simulink model "final_project_dscrt_agmnt"  (R2019b)
settings: Solver=FixedStepAuto  StartTime=0.0  StopTime=10.0  FixedStep=0.01  RelTol=1e-3
undefined symbols (not defined in the file or in its folder): DiscIntNeverNeededParam
libraries: fuzblock x3, simulink x1
settings Model: Creator=Mertcan  LastModifiedBy=Mertcan

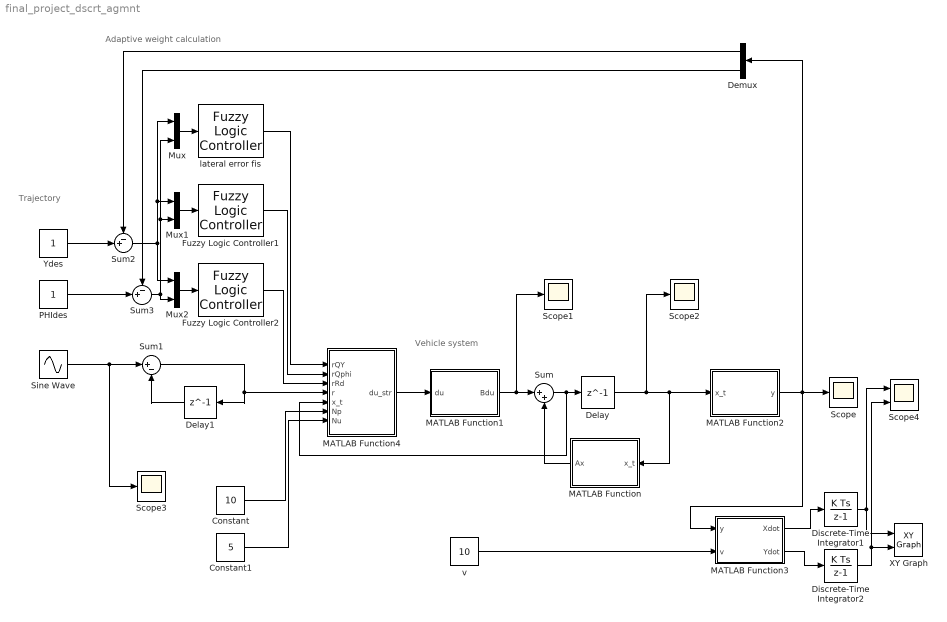
== system final_project_dscrt_agmnt ==
  note: Trajectory
  note: Vehicle system
  note: Adaptive weight calculation
  Constant : Constant  Value=10
  Constant1 : Constant  Value=5
  Delay : Delay  DelayLength=1  SampleTime=0.01
  Delay1 : Delay  DelayLength=1  SampleTime=0.01
  Demux : Demux  Outputs=2
  Discrete-Time Integrator1 : DiscreteIntegrator  SampleTime=0.01  ICPrevOutput=DiscIntNeverNeededParam  ICPrevScaledInput=DiscIntNeverNeededParam
  Discrete-Time Integrator2 : DiscreteIntegrator  SampleTime=0.01  ICPrevOutput=DiscIntNeverNeededParam  ICPrevScaledInput=DiscIntNeverNeededParam
  Fuzzy Logic Controller1 : fuzblock/Fuzzy Logic  Controller  FIS='head_err_surf.fis'  OutputSampleNumber=101  DataType=double  FuzzifiedInputs=off  RuleFiringStrengths=off  RuleOutputs=off  AggregatedOutputs=off  SimulateUsing=Interpreted execution  OutOfRangeInputValueMessage=warning  NoRuleFiredMessage=warning  EmptyOutputFuzzySetMessage=warning
  Fuzzy Logic Controller2 : fuzblock/Fuzzy Logic  Controller  FIS='ang_inc_fw.fis'  OutputSampleNumber=101  DataType=double  FuzzifiedInputs=off  RuleFiringStrengths=off  RuleOutputs=off  AggregatedOutputs=off  SimulateUsing=Interpreted execution  OutOfRangeInputValueMessage=warning  NoRuleFiredMessage=warning  EmptyOutputFuzzySetMessage=warning
  MATLAB Function : MATLAB Function  TreatAsAtomicUnit=on
  MATLAB Function1 : MATLAB Function  TreatAsAtomicUnit=on
  MATLAB Function2 : MATLAB Function  TreatAsAtomicUnit=on
  MATLAB Function3 : MATLAB Function  TreatAsAtomicUnit=on
  MATLAB Function4 : MATLAB Function  TreatAsAtomicUnit=on
  Mux : Mux  Inputs=2
  Mux1 : Mux  Inputs=2
  Mux2 : Mux  Inputs=2
  PHIdes : Constant
  Scope{,1..3} (4 alike) : Scope
  Scope4 : Scope  NumInputPorts=2
  Sine Wave : Sin  Amplitude=0.07  SampleTime=0.01
  Sum : Sum  Inputs=|++
  Sum1 : Sum  Inputs=|+-
  Sum2 : Sum  Inputs=-+|
  Sum3 : Sum  Inputs=-+|
  XY Graph : simulink/Sinks/XY Graph  xmin=-1  xmax=100  ymin=-10  ymax=30  st=-1
  Ydes : Constant
  lateral error fis : fuzblock/Fuzzy Logic  Controller  FIS='lat_err.fis'  OutputSampleNumber=101  DataType=double  FuzzifiedInputs=off  RuleFiringStrengths=off  RuleOutputs=off  AggregatedOutputs=off  SimulateUsing=Interpreted execution  OutOfRangeInputValueMessage=warning  NoRuleFiredMessage=warning  EmptyOutputFuzzySetMessage=warning
  v : Constant  Value=10
  wires:
  MATLAB Function/1(Ax) -> Sum/2
  MATLAB Function1/1(Bdu) -> Scope1/1, Sum/1
  Sum/1 -> MATLAB Function4/5(x_t), Delay/1
  Sine Wave/1 -> Sum1/1, Scope3/1
  v/1 -> MATLAB Function3/2(v)
  MATLAB Function2/1(y) -> Demux/1, MATLAB Function3/1(y), Scope/1
  Discrete-Time Integrator1/1 -> Scope4/1, XY Graph/1
  Discrete-Time Integrator2/1 -> Scope4/2, XY Graph/2
  MATLAB Function3/1(Xdot) -> Discrete-Time Integrator1/1
  MATLAB Function3/2(Ydot) -> Discrete-Time Integrator2/1
  Delay/1 -> Scope2/1, MATLAB Function2/1(x_t), MATLAB Function/1(x_t)
  Sum1/1 -> Delay1/1, MATLAB Function4/4(r)
  Delay1/1 -> Sum1/2
  MATLAB Function4/1(du_str) -> MATLAB Function1/1(du)
  Constant/1 -> MATLAB Function4/6(Np)
  Constant1/1 -> MATLAB Function4/7(Nu)
  Ydes/1 -> Sum2/2
  PHIdes/1 -> Sum3/2
  Demux/1 -> Sum2/1
  Demux/2 -> Sum3/1
  lateral error fis/1 -> MATLAB Function4/1(rQY)
  Fuzzy Logic Controller1/1 -> MATLAB Function4/2(rQphi)
  Fuzzy Logic Controller2/1 -> MATLAB Function4/3(rRd)
  Mux/1 -> lateral error fis/1
  Mux1/1 -> Fuzzy Logic Controller1/1
  Sum3/1 -> Mux2/2, Mux1/2, Mux/2
  Mux2/1 -> Fuzzy Logic Controller2/1
  Sum2/1 -> Mux2/1, Mux1/1, Mux/1

== matlab function final_project_dscrt_agmnt/MATLAB Function1 ==
  data: du input; Bdu output
function Bdu = Bmat(du)

% m = 1350; % kg
% lf = 1.016; % m
% Iz = 4000; % kg.m^2
% Cf = 87594; % N/rad

% dt = 0.1
% B = [0.204160750073782
%     3.22429376254482
%     0.0952067310058050
%     1.74510127293309];

% dt = 0.01

B_k = [0.00308538121733195
    0.601722163601119
    0.00109699431148174
    0.217836958427102];

B_t = [B_k;1];

Bdu = B_t*du;

== matlab function final_project_dscrt_agmnt/MATLAB Function ==
  data: x_t input; Ax output
function Ax = Amat(x_t)

% m = 1350; % kg
% lf = 1.016; % m
% lr = 1.562; % m
% Iz = 4000; % kg.m^2
% Cf = 87594; % N/rad
% Cr = 87594; % N/rad

% dt = 0.1
% A = [1,0.0554395351293068,0,-0.0167590342351909
%     0,0.260529237543850,0,-0.230564952320616
%     0,0.00310316170359759,1,0.0693857231158054
%     0,0.0426922172359289,0,0.452396031479352];

% dt = 0.01

A_k = [1,0.00937715121894016,0,-0.000301547085405976
    0,0.877953203322308,0,-0.0582583895552142
    0,5.58355185705388e-05,1,0.00962808646263230
    0,0.0107873282460033,0,0.926433470211531];
    
B_k = [0.00308538121733195
    0.601722163601119
    0.00109699431148174
    0.217836958427102];

A_t = [A_k, B_k
    zeros(1,4), 1];

Ax = A_t*x_t;

== matlab function final_project_dscrt_agmnt/MATLAB Function2 ==
  data: x_t input; y output
function y = Cmat(x_t)

C_k = [1, 0, 0, 0
    0, 0, 1, 0];

C_t = [C_k, zeros(2,1)];

y = C_t*x_t;

== matlab function final_project_dscrt_agmnt/MATLAB Function3 ==
  data: y input; Xdot output; v input; Ydot output
function [Xdot, Ydot] = CmatXY(y,v)

ydot = y(1);
phi = y(2);

Ydot = sin(phi)*v+cos(phi)*ydot;
Xdot = cos(phi)*v-sin(phi)*ydot;

== matlab function final_project_dscrt_agmnt/MATLAB Function4 ==
  data: rQY input; rQphi input; rRd input; r input; du_str output; x_t input; Np input; Nu input
function du_str = MPC(rQY,rQphi,rRd,r,x_t,Np,Nu)

A_k = [1,0.00937715121894016,0,-0.000301547085405976
    0,0.877953203322308,0,-0.0582583895552142
    0,5.58355185705388e-05,1,0.00962808646263230
    0,0.0107873282460033,0,0.926433470211531];
    
B_k = [0.00308538121733195
    0.601722163601119
    0.00109699431148174
    0.217836958427102];

C_k = [1, 0, 0, 0
    0, 0, 1, 0];

A_t = [A_k, B_k
    zeros(1,4), 1];

B_t = [B_k;1];

C_t = [C_k, zeros(2,1)];

P_t = zeros(2*Np,5);
H_t = zeros(2*Np,Np);
for i = 1:Np
    P_t((2*i-2):(2*i),:) = C_t*A_t^i;
    H_t((2*i-2):(2*i),1) = C_t*A_t^(i-1)*B_t;
    for j = 2:Np
        if (i+j) < (Np+2)
            H_t(2*(i+j-1)-2:2*(i+j-1),j) = H_t((2*i-2):(2*i),1);
        end
    end
end

Q = eye(2*Np);
R = eye(Nu);

M = H_t(:,1:Nu)'*Q*H_t(:,1:Nu)+R;

f = H_t(:,1:Nu)'*Q*(P_t*x_t-r);
    
du = -M\f;

du_str = du(1);
